simulink library "lib"  (R2020a)
settings: Solver=VariableStepAuto  StartTime=0.0  StopTime=10.0  RelTol=1e-3
undefined symbols (not defined in the file or in its folder): sim4Direction, sim4X, sim4Y
libraries: sim3dautolib x1
settings Model: Creator=Matze  LastModifiedBy=Matze

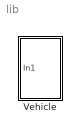
== system lib ==
  Vehicle : Subsystem

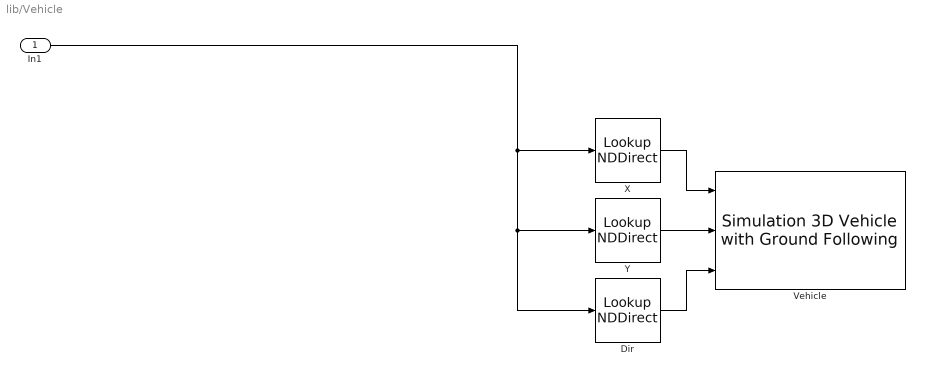
== system lib/Vehicle ==
  In1 : Inport
  Dir : LookupNDDirect  NumberOfTableDimensions=1  Table=sim4Direction
  Vehicle : sim3dautolib/Simulation 3D Vehicle with Ground Following  Priority=-1  PassVehMesh=Sport utility vehicle  VehColor=Orange  InitialPos=[45, 10, 0]  InitialRot=[0, 0, 90]  ActorName=SimulinkVehicle4  SampleTime=-1  ActorType=SimulinkVehicle  ID=4  aMode=3  ActorTag=SimulinkVehicle4  CoordinateScheme=ISO  TransformOutportEnabled=off
      settings: SourceProductBaseCode=DR,VE
  X : LookupNDDirect  NumberOfTableDimensions=1  Table=sim4X
  Y : LookupNDDirect  NumberOfTableDimensions=1  Table=sim4Y
  wires:
  X/1 -> Vehicle/1
  In1/1 -> Dir/1, Y/1, X/1
  Y/1 -> Vehicle/2
  Dir/1 -> Vehicle/3
